simulink model "car_model2"  (Simulink 7.7)
settings: Solver=ode45  StartTime=0.0  StopTime=inf  RelTol=1e-3
libraries: simulink x1, fuzblock x1
settings Model: Creator=piotr  LastModifiedBy=piotr

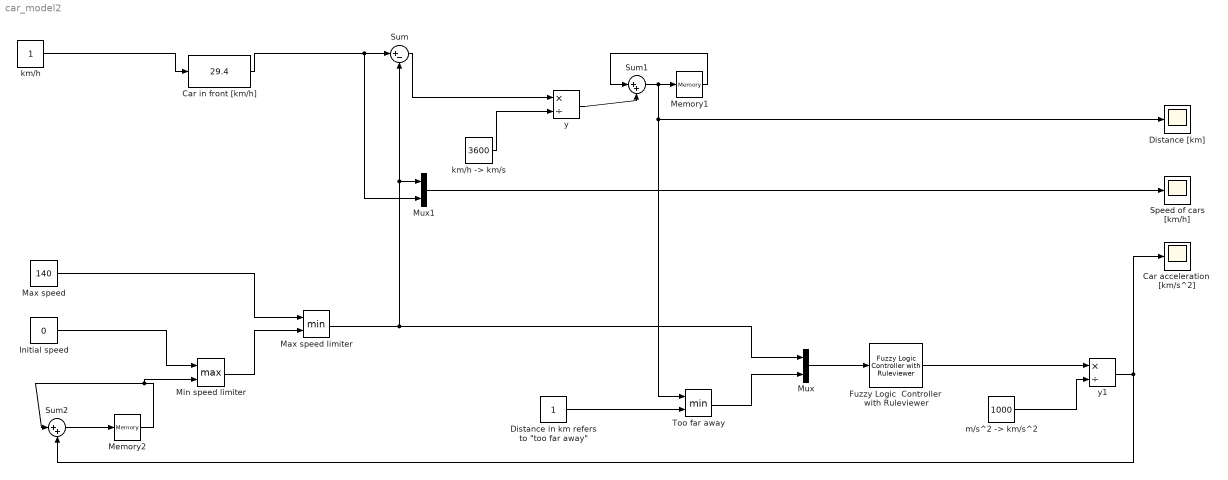
== system car_model2 ==
  Car acceleration  [km/s^2] : Scope
      settings: YMin=0.0088  YMax=0.00891  MaxDataPoints=5000000
  Car in front [km/h] : simulink/Math Operations/Slider Gain  SystemSampleTime=-1  low=0  gain=29.4  high=140
  Distance [km] : Scope
      settings: YMin=-34.015  YMax=-33.9775  SaveName=ScopeData2  MaxDataPoints=5000000
  "Distance in km refers to \"too far away\"" : Constant
  Fuzzy Logic  Controller  with Ruleviewer : fuzblock/Fuzzy Logic  Controller  with Ruleviewer  SystemSampleTime=-1  fismatrix=car2  Ts=1000000
  Initial speed : Constant  Value=0
  Max speed : Constant  Value=140
  Max speed limiter : MinMax  Inputs=2  SampleTime=1
  Memory1 : Memory
  Memory2 : Memory
  Min speed limiter : MinMax  Function=max  Inputs=2  SampleTime=1
  Mux : Mux  Inputs=2
  Mux1 : Mux  Inputs=2
  Speed of cars [km/h] : Scope
      settings: TimeRange=100  YMin=0  YMax=75  MaxDataPoints=5000000
  Sum : Sum  Inputs=|+-
  Sum1 : Sum  Inputs=|++
  Sum2 : Sum  Inputs=|++
  Too far away : MinMax  Inputs=2  SampleTime=1
  km/h : Constant
  "km/h -> km/s" : Constant  Value=3600
  "m/s^2 -> km/s^2" : Constant  Value=1000
  y : Product  Inputs=*/
  y1 : Product  Inputs=*/
  wires:
  km/h/1 -> Car in front [km/h]/1
  Sum1/1 -> Memory1/1, Distance [km]/1, Too far away/1
  Mux1/1 -> Speed of cars [km/h]/1
  Sum/1 -> y/1
  Sum2/1 -> Memory2/1
  Initial speed/1 -> Min speed limiter/1
  Max speed/1 -> Max speed limiter/1
  Min speed limiter/1 -> Max speed limiter/2
  Max speed limiter/1 -> Mux/1, Sum/2, Mux1/1
  "Distance in km refers to \"too far away\""/1 -> Too far away/2
  Memory2/1 -> Sum2/1, Min speed limiter/2
  Memory1/1 -> Sum1/1
  "km/h -> km/s"/1 -> y/2
  Too far away/1 -> Mux/2
  y/1 -> Sum1/2
  Mux/1 -> Fuzzy Logic  Controller  with Ruleviewer/1
  "m/s^2 -> km/s^2"/1 -> y1/2
  y1/1 -> Car acceleration  [km/s^2]/1, Sum2/2
  Fuzzy Logic  Controller  with Ruleviewer/1 -> y1/1
  Car in front [km/h]/1 -> Sum/1, Mux1/2
